simulink model "MODEL"  (Simulink 8.7)
settings: Solver=ode15s  StartTime=0.0  StopTime=100000  RelTol=1e-3
values from neighbouring files (symbols this model uses):
  alfa_ax = -0.3e-5    (= -3e-06)    [INPUT_DATA.m]
  alfa_coolant = -0.3e-5    (= -3e-06)    [INPUT_DATA.m]
  alfa_CRs = 1e-5    (= 1e-05)    [INPUT_DATA.m]
  alfa_rad = -0.3e-5    (= -3e-06)    [INPUT_DATA.m]
  betatot = betatot + beta_i(j)    [INPUT_DATA.m]
  boolean_gamma = 0    [INPUT_DATA.m]    (also in MASSFLOW_RAMP.m = 1)
  boolean_reat = 0    [INPUT_DATA.m]    (also in REACTIVITY_RAMP.m = 1)
  boolean_Tin = 0    [INPUT_DATA.m]
  Ci_eta = 1    [INPUT_DATA.m]
  Ci_psi = 1    [INPUT_DATA.m]
  cp_fuel = 182.63    [INPUT_DATA.m]
  cp_Na = cp_Na_av    [INPUT_DATA.m]
  gamma = potenzatot0/(cp_Na_av*(T_out0-T_in0))    [INPUT_DATA.m]
  K_Doppler = -374e-5    (= -0.00374)    [INPUT_DATA.m]
  Linv = 0.44600E-6    (= 4.46e-07)    [INPUT_DATA.m]
  M_fuel = smear*Vol_fuel*rho_teorica*pin    [INPUT_DATA.m]
  Portata0 = gamma    [INPUT_DATA.m]
  potenzatot0 = 15e6    (= 15000000)    [INPUT_DATA.m]
  risposta1 = 1    [INPUT_DATA.m]    (also in MASSFLOW_RAMP.m = 3; REACTIVITY_RAMP.m)
  slope_gamma = 0    [INPUT_DATA.m]    (also in MASSFLOW_RAMP.m = slope_variazione*gamma)
  slope_reat = 0    [INPUT_DATA.m]    (also in REACTIVITY_RAMP.m = step_reat/tempo_reat)
  slope_Tin = 0    [INPUT_DATA.m]
  step_gamma = 0    [INPUT_DATA.m]    (also in MASSFLOW_RAMP.m = step_variazione; REACTIVITY_RAMP.m)
  step_reat = 0    [INPUT_DATA.m]    (also in REACTIVITY_RAMP.m = input('Insert the reactivity [in pcm] (nominal value = 0) '))
  step_Tin = 0    [INPUT_DATA.m]    (also in REACTIVITY_RAMP.m)
  T_coolant0 = (T_out0 + T_in0)/2    (= 430)    [INPUT_DATA.m]
  T_fuel0 = potenzatot0/U_tot + T_coolant0    [INPUT_DATA.m]
  T_in0 = 410    [INPUT_DATA.m]
  T_out0 = 450    [INPUT_DATA.m]
  tau_fuel = (U_tot/M_fuel/cp_fuel)^-1    [INPUT_DATA.m]
  V_Na = V_Na_core    [INPUT_DATA.m]
undefined symbols (not defined in the file or in its folder): beta_i, lambda_i, ln, U_tot
libraries: simulink x3
settings Model: Creator=sara  LastModifiedBy=danielk5
settings DataIOCC: SignalLoggingSaveFormat=ModelDataLogs
settings OptimizationCC: ExpressionDepthLimit=2147483647  InitFltsAndDblsToZero=on
settings DebuggingCC: SolverPrmCheckMsg=warning  FcnCallInpInsideContextMsg=UseLocalSettings  StateNameClashWarn=warning
settings GRTTargetCC: CombineOutputUpdateFcns=off  GRTInterface=on

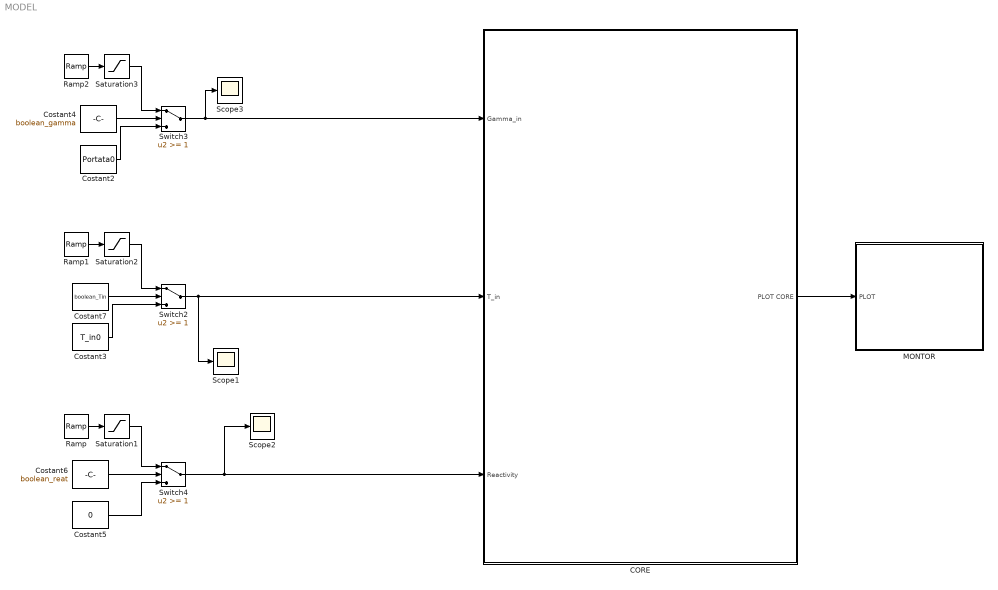
== system MODEL ==
  CORE : Subsystem
  Costant2 : Constant  Value=Portata0
  Costant3 : Constant  Value=T_in0
  Costant4 : Constant  Value=boolean_gamma
  Costant5 : Constant  Value=0
  Costant6 : Constant  Value=boolean_reat
  Costant7 : Constant  Value=boolean_Tin
  MONTOR : Subsystem  Tag=MONITOR
  Ramp : simulink/Sources/Ramp  slope=slope_reat  start=100  X0=0
  Ramp1 : simulink/Sources/Ramp  slope=slope_Tin  start=100  X0=T_in0
  Ramp2 : simulink/Sources/Ramp  slope=slope_gamma  start=100  X0=gamma
  Saturation1 : Saturate  UpperLimit=abs(step_reat)  LowerLimit=-abs(step_reat)  OutMin=-abs(step_reat)  OutMax=abs(step_reat)
  Saturation2 : Saturate  UpperLimit=T_in0+abs(step_Tin)  LowerLimit=T_in0-abs(step_Tin)  OutMin=T_in0-abs(step_Tin)  OutMax=T_in0+abs(step_Tin)
  Saturation3 : Saturate  UpperLimit=gamma+abs(step_gamma*gamma)  LowerLimit=gamma-abs(step_gamma*gamma)  OutMin=gamma-abs(step_gamma*gamma)  OutMax=gamma+abs(step_gamma*gamma)
  Scope1 : Scope
  Scope2 : Scope
  Scope3 : Scope
  Switch2 : Switch  Threshold=1
  Switch3 : Switch  Threshold=1
  Switch4 : Switch  Threshold=1
  wires:
  Costant2/1 -> Switch3/3
  Costant4/1 -> Switch3/2
  Saturation3/1 -> Switch3/1
  Ramp2/1 -> Saturation3/1
  Switch3/1 -> CORE/1(Gamma_in), Scope3/1
  Switch2/1 -> CORE/2(T_in), Scope1/1
  CORE/1(PLOT CORE) -> MONTOR/1(PLOT)
  Saturation2/1 -> Switch2/1
  Costant3/1 -> Switch2/3
  Costant7/1 -> Switch2/2
  Ramp1/1 -> Saturation2/1
  Saturation1/1 -> Switch4/1
  Costant5/1 -> Switch4/3
  Costant6/1 -> Switch4/2
  Ramp/1 -> Saturation1/1
  Switch4/1 -> Scope2/1, CORE/3(Reactivity)

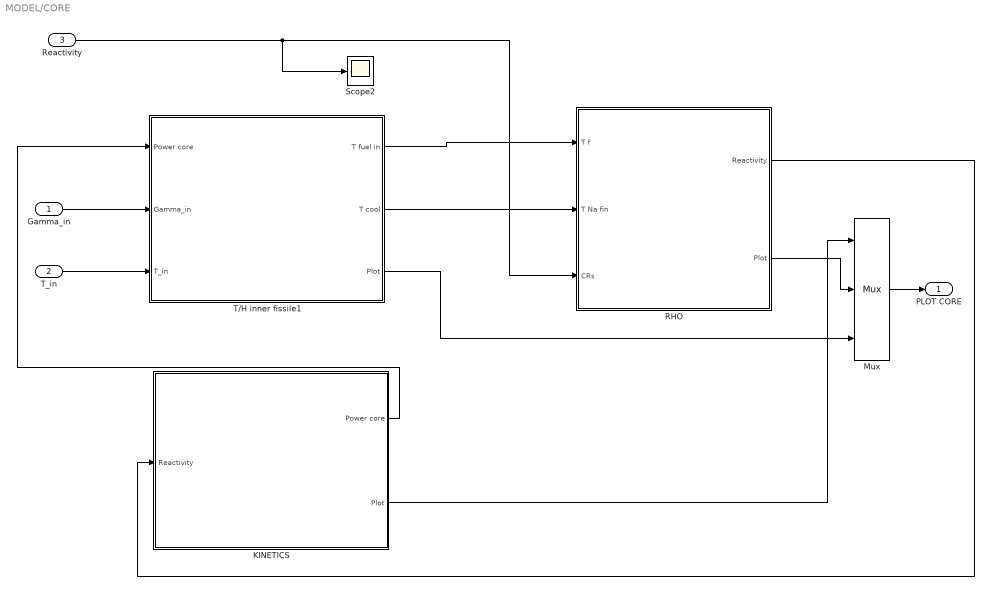
== system MODEL/CORE ==
  Gamma_in : Inport
  T_in : Inport  Port=2
  Reactivity : Inport  Port=3
  KINETICS : Subsystem
  Mux : Mux  Inputs=3
  RHO : Subsystem
  Scope2 : Scope
  T/H inner fissile1 : Subsystem
  PLOT CORE : Outport
  wires:
  Gamma_in/1 -> T/H inner fissile1/2(Gamma_in)
  T_in/1 -> T/H inner fissile1/3(T_in)
  Mux/1 -> PLOT CORE/1
  KINETICS/2(Plot) -> Mux/1
  Reactivity/1 -> RHO/3(CRs), Scope2/1
  T/H inner fissile1/3(Plot) -> Mux/3
  RHO/2(Plot) -> Mux/2
  RHO/1(Reactivity) -> KINETICS/1(Reactivity)
  KINETICS/1(Power core) -> T/H inner fissile1/1(Power core)
  T/H inner fissile1/1(T fuel in) -> RHO/1(T f)
  T/H inner fissile1/2(T cool) -> RHO/2(T Na fin)

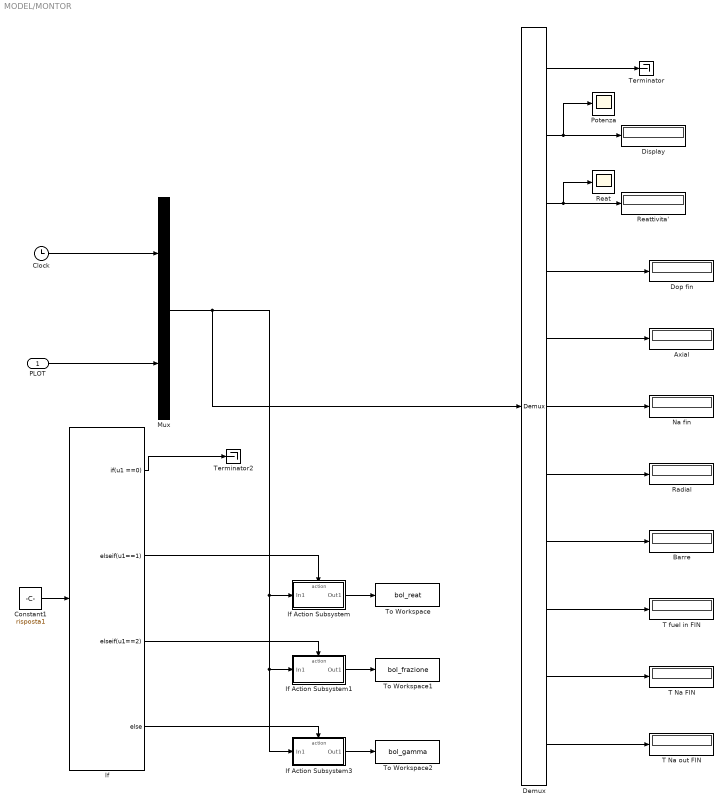
== system MODEL/MONTOR ==
  PLOT : Inport
  Axial : Display
  Barre : Display
  Clock : Clock
  Constant1 : Constant  Value=risposta1
  Demux : Demux  Outputs=11
  Display : Display
  Dop fin : Display
  If : If  IfExpression=u1 ==0  ElseIfExpressions=u1==1,u1==2
  If Action Subsystem : Subsystem  TreatAsAtomicUnit=on
  If Action Subsystem1 : Subsystem  TreatAsAtomicUnit=on
  If Action Subsystem3 : Subsystem  TreatAsAtomicUnit=on
  Mux : Mux  Inputs=2
  Na fin : Display
  Potenza : Scope
  Radial : Display
  Reat : Scope
  Reattivita' : Display
  T Na FIN : Display
  T Na out FIN : Display
  T fuel in FIN : Display
  Terminator : Terminator
  Terminator2 : Terminator
  To Workspace : ToWorkspace  VariableName=bol_reat  SampleTime=-1
  To Workspace1 : ToWorkspace  VariableName=bol_frazione  SampleTime=-1
  To Workspace2 : ToWorkspace  VariableName=bol_gamma  SampleTime=-1
  wires:
  Mux/1 -> If Action Subsystem/1(In1), If Action Subsystem3/1(In1), If Action Subsystem1/1(In1), Demux/1
  Clock/1 -> Mux/1
  PLOT/1 -> Mux/2
  Demux/1 -> Terminator/1
  Constant1/1 -> If/1
  If/1 -> Terminator2/1
  If/2 -> If Action Subsystem/Action
  If Action Subsystem/1(Out1) -> To Workspace/1
  If Action Subsystem1/1(Out1) -> To Workspace1/1
  If Action Subsystem3/1(Out1) -> To Workspace2/1
  Demux/4 -> Dop fin/1
  Demux/5 -> Axial/1
  Demux/6 -> Na fin/1
  Demux/7 -> Radial/1
  Demux/8 -> Barre/1
  If/3 -> If Action Subsystem1/Action
  If/4 -> If Action Subsystem3/Action
  Demux/3 -> Reat/1, Reattivita'/1
  Demux/2 -> Potenza/1, Display/1
  Demux/9 -> T fuel in FIN/1
  Demux/10 -> T Na FIN/1
  Demux/11 -> T Na out FIN/1

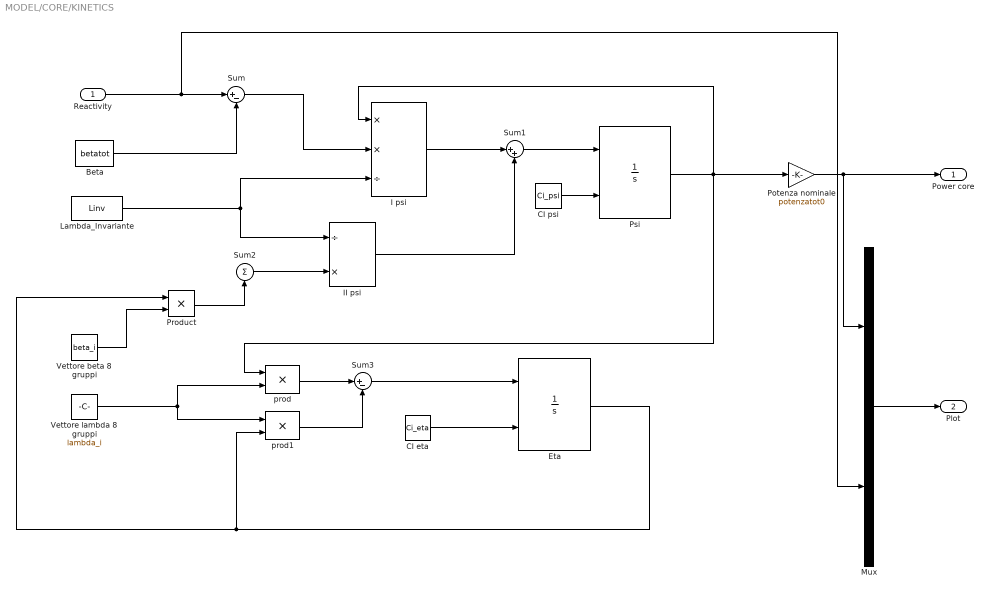
== system MODEL/CORE/KINETICS ==
  Reactivity : Inport
  Beta : Constant  Value=betatot
  CI eta : Constant  Value=Ci_eta
  CI psi : Constant  Value=Ci_psi
  Eta : Integrator  InitialConditionSource=external
  I psi : Product  Inputs=**/  RndMeth=Zero
  II psi : Product  Inputs=/*  RndMeth=Zero
  Lambda_Invariante : Constant  Value=Linv
  Mux : Mux  Inputs=2
  Potenza nominale : Gain  Gain=potenzatot0
  Product : Product  RndMeth=Zero
  Psi : Integrator  InitialConditionSource=external
  Sum : Sum  Inputs=|+-
  Sum1 : Sum  Inputs=|++
  Sum2 : Sum  Inputs=|+
  Sum3 : Sum  Inputs=|+-
  Vettore beta 8 gruppi : Constant  Value=beta_i
  Vettore lambda 8 gruppi : Constant  Value=lambda_i
  prod : Product  Inputs=**  RndMeth=Zero
  prod1 : Product  Inputs=**  RndMeth=Zero
  Power core : Outport
  Plot : Outport  Port=2
  wires:
  Beta/1 -> Sum/2
  Lambda_Invariante/1 -> I psi/3, II psi/1
  Sum/1 -> I psi/2
  I psi/1 -> Sum1/1
  Sum1/1 -> Psi/1
  CI psi/1 -> Psi/2
  Psi/1 -> I psi/1, prod/1, Potenza nominale/1
  Potenza nominale/1 -> Power core/1, Mux/1
  Vettore beta 8 gruppi/1 -> Product/2
  Product/1 -> Sum2/1
  Sum2/1 -> II psi/2
  II psi/1 -> Sum1/2
  prod/1 -> Sum3/1
  prod1/1 -> Sum3/2
  Sum3/1 -> Eta/1
  CI eta/1 -> Eta/2
  Eta/1 -> Product/1, prod1/2
  Vettore lambda 8 gruppi/1 -> prod/2, prod1/1
  Mux/1 -> Plot/1
  Reactivity/1 -> Mux/2, Sum/1

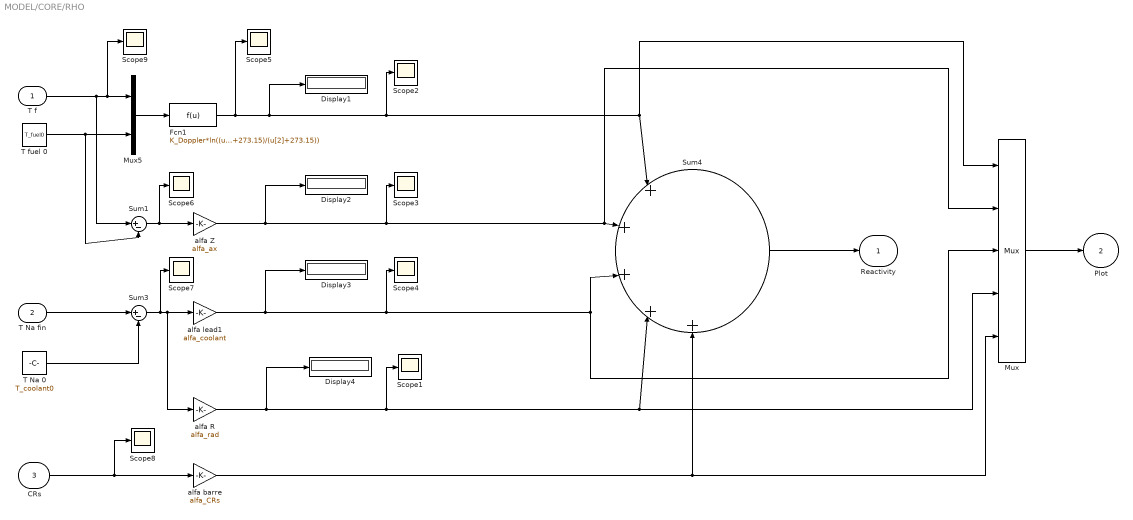
== system MODEL/CORE/RHO ==
  T f : Inport
  T Na fin : Inport  Port=2
  CRs : Inport  Port=3
  Display{1..4} (4 alike) : Display
  Fcn1 : Fcn  Expr=K_Doppler*ln((u[1]+273.15)/(u[2]+273.15))
  Mux : Mux  Inputs=5
  Mux5 : Mux  Inputs=2
  Scope{1..9} (9 alike) : Scope
  Sum1 : Sum  Inputs=|+-
  Sum3 : Sum  Inputs=|+-
  Sum4 : Sum  Inputs=|+++++
  "T Na 0 " : Constant  Value=T_coolant0
  T fuel 0 : Constant  Value=T_fuel0
  alfa R : Gain  Gain=alfa_rad
  alfa Z : Gain  Gain=alfa_ax
  alfa barre : Gain  Gain=alfa_CRs
  alfa lead1 : Gain  Gain=alfa_coolant
  Reactivity : Outport
  Plot : Outport  Port=2
  wires:
  CRs/1 -> Scope8/1, alfa barre/1
  Mux/1 -> Plot/1
  T f/1 -> Sum1/1, Scope9/1, Mux5/1
  Mux5/1 -> Fcn1/1
  T Na fin/1 -> Sum3/1
  "T Na 0 "/1 -> Sum3/2
  Sum4/1 -> Reactivity/1
  T fuel 0/1 -> Mux5/2, Sum1/2
  Sum1/1 -> Scope6/1, alfa Z/1
  Fcn1/1 -> Scope5/1, Display1/1, Scope2/1, Sum4/1, Mux/1
  Sum3/1 -> Scope7/1, alfa R/1, alfa lead1/1
  alfa Z/1 -> Display2/1, Scope3/1, Mux/2, Sum4/2
  alfa lead1/1 -> Display3/1, Scope4/1, Sum4/3, Mux/3
  alfa R/1 -> Display4/1, Mux/4, Sum4/4, Scope1/1
  alfa barre/1 -> Mux/5, Sum4/5

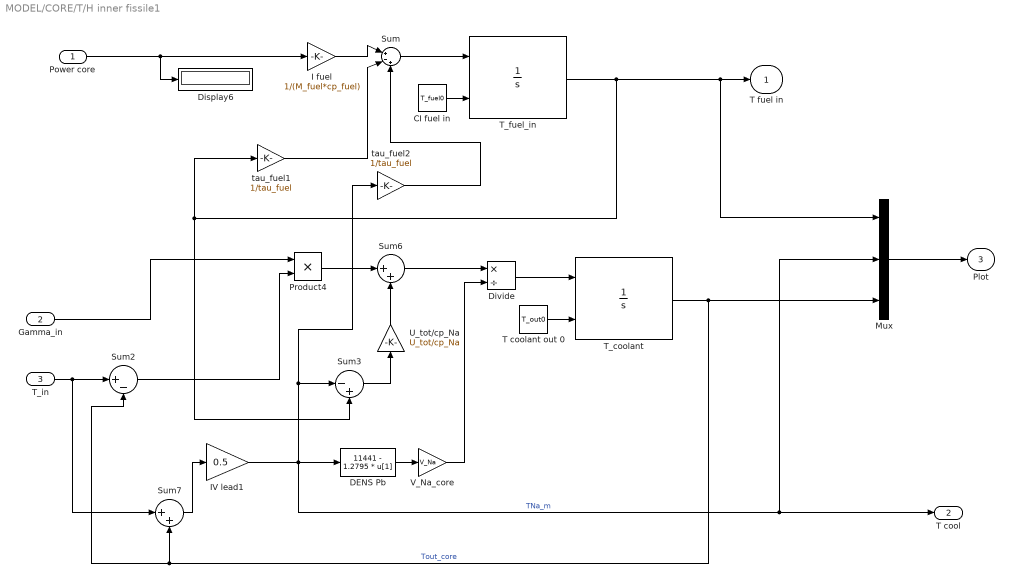
== system MODEL/CORE/T/H inner fissile1 ==
  Power core : Inport
  Gamma_in : Inport  Port=2
  T_in : Inport  Port=3
  CI fuel in : Constant  Value=T_fuel0
  DENS Pb : Fcn  Expr=11441 - 1.2795 * u[1]
  Display6 : Display
  Divide : Product  Inputs=*/
  I fuel : Gain  Gain=1/(M_fuel*cp_fuel)
  IV lead1 : Gain  Gain=0.5
  Mux : Mux  Inputs=3
  Product4 : Product  RndMeth=Zero
  Sum : Sum  Inputs=|+-+
  Sum2 : Sum  Inputs=|+-
  Sum3 : Sum  Inputs=|-+
  Sum6 : Sum  Inputs=|++
  Sum7 : Sum  Inputs=|++
  T coolant out 0 : Constant  Value=T_out0
  T_coolant : Integrator  InitialConditionSource=external
  T_fuel_in : Integrator  InitialConditionSource=external
  U_tot/cp_Na : Gain  Gain=U_tot/cp_Na
  V_Na_core : Gain  Gain=V_Na
  tau_fuel1 : Gain  Gain=1/tau_fuel
  tau_fuel2 : Gain  Gain=1/tau_fuel
  T fuel in : Outport
  T cool : Outport  Port=2
  Plot : Outport  Port=3
  wires:
  Power core/1 -> I fuel/1, Display6/1
  I fuel/1 -> Sum/1
  tau_fuel1/1 -> Sum/2
  Sum/1 -> T_fuel_in/1
  CI fuel in/1 -> T_fuel_in/2
  tau_fuel2/1 -> Sum/3
  Mux/1 -> Plot/1
  T coolant out 0/1 -> T_coolant/2
  DENS Pb/1 -> V_Na_core/1
  V_Na_core/1 -> Divide/2
  Divide/1 -> T_coolant/1
  Sum6/1 -> Divide/1
  Product4/1 -> Sum6/1
  Gamma_in/1 -> Product4/1
  Sum2/1 -> Product4/2
  T_in/1 -> Sum2/1, Sum7/1
  T_coolant/1 -> Sum2/2, Sum7/2, Mux/3  "Tout_core"
  Sum7/1 -> IV lead1/1
  IV lead1/1 -> tau_fuel2/1, Sum3/1, DENS Pb/1, Mux/2, T cool/1  "TNa_m"
  Sum3/1 -> U_tot/cp_Na/1
  U_tot/cp_Na/1 -> Sum6/2
  T_fuel_in/1 -> tau_fuel1/1, Sum3/2, Mux/1, T fuel in/1

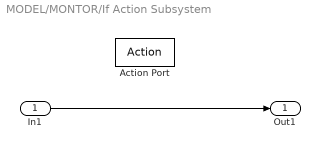
== system MODEL/MONTOR/If Action Subsystem ==
  In1 : Inport
  Action Port : ActionPort  ActionType=elseif
  Out1 : Outport
  wires:
  In1/1 -> Out1/1

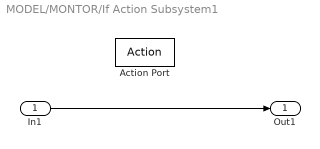
== system MODEL/MONTOR/If Action Subsystem1 ==
  In1 : Inport
  Action Port : ActionPort  ActionType=elseif
  Out1 : Outport
  wires:
  In1/1 -> Out1/1

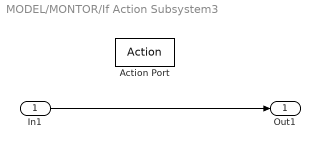
== system MODEL/MONTOR/If Action Subsystem3 ==
  In1 : Inport
  Action Port : ActionPort  ActionType=else
  Out1 : Outport
  wires:
  In1/1 -> Out1/1
